simulink model "untitled2"  (R2018a)
settings: Solver=ode45  StartTime=0.0  StopTime=10  RelTol=1e-3
settings Model: Creator=HLY  LastModifiedBy=14223
settings CodeAppCC: StateflowObjectComments=on

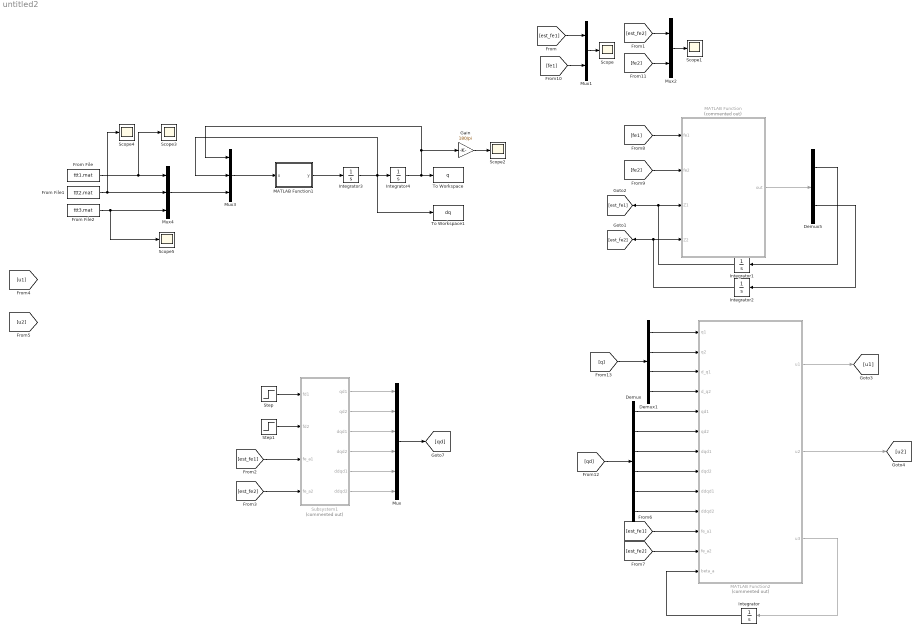
== system untitled2 ==
  Demux : Demux  Outputs=6
  Demux1 : Demux
  Demux5 : Demux  Outputs=[1;1]
  From File : FromFile  FileName=ttt1.mat  OutDataTypeStr=double
  From File1 : FromFile  FileName=ttt2.mat  OutDataTypeStr=double
  From File2 : FromFile  FileName=ttt3.mat  OutDataTypeStr=double
  Gain : Gain  Gain=180/pi
  Integrator : Integrator
  Integrator1 : Integrator
  Integrator2 : Integrator
  Integrator3 : Integrator  InitialCondition=[0 0 0]
  Integrator4 : Integrator  InitialCondition=[0 0 0]
  MATLAB Function : MATLAB Function  Commented=on  TreatAsAtomicUnit=on
  MATLAB Function1 : MATLAB Function  TreatAsAtomicUnit=on
  MATLAB Function2 : MATLAB Function  Commented=on  TreatAsAtomicUnit=on
  Mux : Mux  Inputs=6
  Mux1 : Mux  Inputs=2
  Mux2 : Mux  Inputs=2
  Mux3 : Mux  Inputs=3
  Mux4 : Mux  Inputs=3
  Scope{,1..5} (6 alike) : Scope
  Step : Step  After=10  SampleTime=0
  Step1 : Step  After=10  SampleTime=0
  Subsystem1 : Subsystem  Commented=on
  To Workspace : ToWorkspace  VariableName=q  SampleTime=-1
  To Workspace1 : ToWorkspace  VariableName=dq  SampleTime=-1
  wires:
  MATLAB Function/1(out) -> Demux5/1
  Demux5/1 -> Integrator1/1
  Demux5/2 -> Integrator2/1
  [est_fe1] -> Mux1/1
  [est_fe2] -> Mux2/1
  Mux1/1 -> Scope/1
  Mux2/1 -> Scope1/1
  MATLAB Function2/1(u1) -> [u1]
  MATLAB Function2/2(u2) -> [u2]
  Integrator/1 -> MATLAB Function2/13(beta_a)
  MATLAB Function2/3(u3) -> Integrator/1
  Integrator1/1 -> MATLAB Function/3(Z1), [est_fe1]
  Integrator2/1 -> MATLAB Function/4(Z2), [est_fe2]
  Step/1 -> Subsystem1/1(fd1)
  Step1/1 -> Subsystem1/2(fd2)
  [est_fe1] -> Subsystem1/3(fe_a1)
  [est_fe2] -> Subsystem1/4(fe_a2)
  [est_fe1] -> MATLAB Function2/11(fe_a1)
  [est_fe2] -> MATLAB Function2/12(fe_a2)
  [fe2] -> MATLAB Function/2(fe2)
  [fe1] -> MATLAB Function/1(fe1)
  [fe1] -> Mux1/2
  [fe2] -> Mux2/2
  Mux/1 -> [qd]
  Subsystem1/1(qd1) -> Mux/1
  Subsystem1/2(qd2) -> Mux/2
  Subsystem1/3(dqd1) -> Mux/3
  Subsystem1/4(dqd2) -> Mux/4
  Subsystem1/5(ddqd1) -> Mux/5
  Subsystem1/6(ddqd2) -> Mux/6
  Demux/1 -> MATLAB Function2/5(qd1)
  Demux/2 -> MATLAB Function2/6(qd2)
  Demux/3 -> MATLAB Function2/7(dqd1)
  Demux/4 -> MATLAB Function2/8(dqd2)
  Demux/5 -> MATLAB Function2/9(ddqd1)
  Demux/6 -> MATLAB Function2/10(ddqd2)
  [qd] -> Demux/1
  [q] -> Demux1/1
  Demux1/4 -> MATLAB Function2/4(d_q2)
  Demux1/1 -> MATLAB Function2/1(q1)
  Demux1/2 -> MATLAB Function2/2(q2)
  Demux1/3 -> MATLAB Function2/3(d_q1)
  Gain/1 -> Scope2/1
  From File1/1 -> Scope4/1, Mux4/2
  Mux3/1 -> MATLAB Function1/1(u)
  Mux4/1 -> Mux3/3
  From File2/1 -> Scope5/1, Mux4/3
  Integrator4/1 -> Gain/1, Mux3/1, To Workspace/1
  MATLAB Function1/1(y) -> Integrator3/1
  Integrator3/1 -> To Workspace1/1, Mux3/2, Integrator4/1
  From File/1 -> Scope3/1, Mux4/1

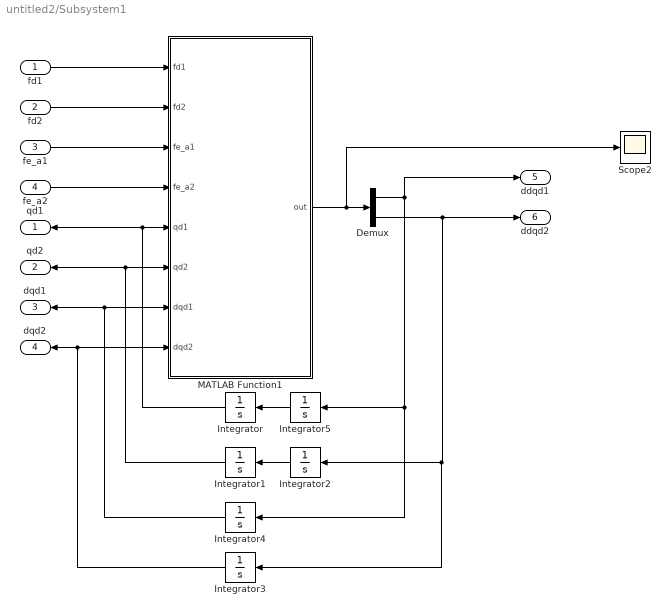
== system untitled2/Subsystem1 ==
  fd1 : Inport
  fd2 : Inport  Port=2
  fe_a1 : Inport  Port=3
  fe_a2 : Inport  Port=4
  Demux : Demux  Outputs=2
  Integrator : Integrator  InitialCondition=0.483
  Integrator1 : Integrator  InitialCondition=0.684
  Integrator{2..5} (4 alike) : Integrator
  MATLAB Function1 : MATLAB Function  TreatAsAtomicUnit=on
  Scope2 : Scope
  qd1 : Outport
  qd2 : Outport  Port=2
  dqd1 : Outport  Port=3
  dqd2 : Outport  Port=4
  ddqd1 : Outport  Port=5
  ddqd2 : Outport  Port=6
  wires:
  MATLAB Function1/1(out) -> Scope2/1, Demux/1
  fd1/1 -> MATLAB Function1/1(fd1)
  fd2/1 -> MATLAB Function1/2(fd2)
  fe_a1/1 -> MATLAB Function1/3(fe_a1)
  fe_a2/1 -> MATLAB Function1/4(fe_a2)
  Integrator/1 -> qd1/1, MATLAB Function1/5(qd1)
  Integrator5/1 -> Integrator/1
  Integrator2/1 -> Integrator1/1
  Integrator1/1 -> MATLAB Function1/6(qd2), qd2/1
  Integrator4/1 -> MATLAB Function1/7(dqd1), dqd1/1
  Integrator3/1 -> dqd2/1, MATLAB Function1/8(dqd2)
  Demux/1 -> Integrator5/1, Integrator4/1, ddqd1/1
  Demux/2 -> Integrator3/1, Integrator2/1, ddqd2/1

== matlab function untitled2/MATLAB Function1 ==
  data: u input; y output
function y = fcn(u)
a1=0.02;a2=0.475;a3=0.02;g=9.81;
q0=u(1);q1=u(2);q2=u(3);
dq0=u(4);dq1=u(5);dq2=u(6);
tol1=u(7);tol2=u(8);tol3=u(9);
I1xx=0;I1xy=0;I1xz=0;I1yyc=0;I1yz=0;I1zzc=0.5;
l1x=0.5*a1;l1y=0;l1z=0;
m1=12;
rlx=l1x/m1;
I1yy=m1*(rlx^2);%平行轴定理
I1zz=I1zzc+m1*(rlx^2);
I2xx=0;I2xy=0;I2xz=0;I2yyc=0;I2yz=0;I2zzc=0.2;
l2x=0.5*a2;l2y=0;l2z=0;
m2=8;
r2x=l2x/m2;
I2yy=m2*(r2x^2);
I2zz=I2zzc+m2*(r2x^2);
I3xx=0;I3xy=0;I3xz=0;I3yyc=0;I3yz=0;I3zzc=0.1;
l3x=0.5*a3;l3y=0;l3z=0;
m3=5;
r3x=l3x/m3;
I3yy=m3*(r3x^2);
I3zz=I3zzc+m3*(r3x^2);
F1s=97.26;F1v=96.14;F2s=1.03;F2v=65.03;F3s=33.43;F3v=19.3;
%F1s= 90;F1v=96.14;F2s=0;F2v=65.03;F3s=30;F3v=19.3;

 Xmin=[I1zz+I2yy+I3yy+m2*a1^2+m3*(a1^2+a2^2);I2xx-I2yy-m3*a2^2;I2xy;I2xz-a2*l3z;I2yz;I2zz+m3*a2^2;l2x+m3*a2;l2y;I3xx-I3yy;I3xy;I3xz;I3yz;I3zz;l3x;l3y;F1s;F1v;F2s;F2v;F3s;F3v];
 Xmin=[I1zz+I2yy+I3yy+m2*a1^2+m3*(a1^2+a2^2);I2xx-I2yy-m3*a2^2;I2xy;I2xz-a2*l3z;I2yz;I2zz+m3*a2^2;l2x+m3*a2;l2y;I3xx-I3yy;I3xy;I3xz;I3yz;I3zz;l3x;l3y;F1s;F1v;F2s;F2v;F3s;F3v];
 m11=Xmin(1)+(cos(q1)^2)*Xmin(2)-sin(2*q1)*Xmin(3)+2*a1*sin(q1)*Xmin(7)+2*a1*cos(q1)*Xmin(8)+(1/2+cos(2*q1+2*q2)/2)* Xmin(9)-sin(2*(q1+q2))*Xmin(10)+(a2.*cos(q2)+2*a1.*sin(q1+q2)-a2*cos(2*q1+q2))*Xmin(14)+(a2*sin(2*q1+q2)-a2*sin(q2)+2*a1*cos(q1+q2))*Xmin(15);
 m12=cos(q1)*Xmin(4)-sin(q1)*Xmin(5)+cos(q1+q2)*Xmin(11)-sin(q1+q2)*Xmin(12);
 m13=cos(q1+q2)*Xmin(11)-sin(q1+q2)*Xmin(12);
 m21=cos(q1)*Xmin(4)+cos(q1+q2)*Xmin(11)-sin(q1+q2)*Xmin(12);
 m22=Xmin(6)+Xmin(13)+2*a2.*cos(q2)*Xmin(14)- 2*a2*sin(q2)*Xmin(15);
 m23=Xmin(13)+a2*cos(q2)*Xmin(14)-2*a2*sin(q2)*Xmin(15);
 m31=cos(q1+q2)*Xmin(11)-sin(q1+q2)*Xmin(12);
 m32=Xmin(13)+a2*cos(q2)*Xmin(14)-a2*sin(q2)*Xmin(15);
 m33=Xmin(13);
 c1= -cos(q1).*2.*dq0.*dq1.*sin(q1)*Xmin(2)-2*dq0.*dq1.*cos(2*q1).*Xmin(3)-dq1.^2.*sin(q1)*Xmin(4)-(dq1.^2).*cos(q1)*Xmin(5)+2*a1*dq0.*dq1.*cos(q1)*Xmin(7)-2*a1*dq0.*dq1.*sin(q1)*Xmin(8)-(dq0.*dq1.*sin(2*q1+2*q2)+dq0.*dq2.*sin(2*q1+2*q2))*Xmin(9)-2*dq0.*(dq1+dq2).*cos(2*(q1+q2))*Xmin(10)-(sin(q1+q2).*dq1.^2+2*sin(q1+q2).*dq1.*dq2+sin(q1+q2).*dq2.^2)*Xmin(11)+...
    -((dq1+dq2).^2).*cos(q1+q2)*Xmin(12)+(2*a1*dq0.*dq1.*cos(q1+q2)+2*a1*dq0.*dq2.*cos(q1+q2)-a2*dq0.*dq2.*sin(q2)+2*a2*dq0.*dq1.*sin(2*q1+q2)+a2*dq0.*dq2.*sin(2*q1+q2))*Xmin(14)+(-2*a1*dq0.*dq1.*sin(q1+q2)-2*a1*dq0.*dq2.*sin(q1+q2)-a2*dq0.*dq2.*cos(q2)+2*a2*dq0.*dq1.*cos(2*q1+q2)+a2*dq0.*dq2.*cos(2*q1+q2))*Xmin(15);
 c2=(dq0.^2).*cos(q1).*sin(q1)*Xmin(2)+(dq0.^2).*cos(2*q1)*Xmin(3)-a1*(dq0.^2).*cos(q1)*Xmin(7)+a1*(dq0.^2).*sin(q1)*Xmin(8)+((dq0.^2).*sin(2*(q1+q2)))/2*Xmin(9)+(dq0.^2).*cos(2*(q1+q2))*Xmin(10)+(-a1*dq0.^2.*cos(q1+q2)-a2*dq2.^2.*sin(q2)-a2*dq0.^2.*sin(2*q1+q2)-2*a2*dq1.*dq2.*sin(q2))*Xmin(14)+(a1*dq0.^2.*sin(q1+q2)-a2*dq2.^2.*cos(q2)-a2*dq0.^2.*cos(2*q1+q2)-2*a2*dq1.*dq2.*cos(q2))*Xmin(15);
 c3=0.5*dq0.^2.*sin(2*(q1+q2))*Xmin(9)+dq0.^2.*cos(2*(q1+q2))*Xmin(10)+(cos(q2).*(a2*(-cos(q1)).*sin(q1).*dq0.^2-a1*dq0.^2.*cos(q1))-sin(q2).*(-a2.*(dq0.^2.*sin(q1).^2+dq1.^2)-a1*dq0.^2.*sin(q1)))*Xmin(14)+...
    +(-sin(q2).*(a2*(-cos(q1).*sin(q1).*dq0.^2)-a1*dq0.^2.*cos(q1))-cos(q2).*(-a2.*(dq0.^2.*sin(q1).^2+dq1.^2)-a1*dq0.^2.*sin(q1)))*Xmin(15);
 g1=0;
 g2=(-g*sin(q1)*Xmin(7)-g*cos(q1)*Xmin(8)-g*sin(q1+q2)*Xmin(14)-g*cos(q1+q2)*Xmin(15));
 g3=(-g*(sin(q1)*cos(q2)+sin(q2)*cos(q1))*Xmin(14)- g*(-sin(q1)*sin(q2)+cos(q1)*cos(q1))*Xmin(15));
 f1=sign(dq0)*Xmin(16)+dq0*Xmin(17);
 f2=sign(dq1)*Xmin(18)+dq1*Xmin(19);
 f3=sign(dq2)*Xmin(20)+dq2*Xmin(21);
 M=[m11,m12,m13;m21,m22,m23;m31,m32,m33];C=[c1;c2;c3];G=[g1;g2;g3];f=[f1;f2;f3];tol=[tol1;tol2;tol3];
 ddq=inv(M)*(tol-C-G-f);
 y=ddq;
end

== matlab function untitled2/MATLAB Function ==
  data: out output; fe1 input; fe2 input; Z1 input; Z2 input
function out=Est_contactforce(fe1,fe2,Z1,Z2)
L=[50 0;0 50];
Fe=[fe1;fe2];
%Fe=Ke*(X-Xe);
Z=[Z1;Z2];
dEst_Fe=L*(Fe-Z);
out=dEst_Fe;

== matlab function untitled2/MATLAB Function2 ==
  data: q1 input; q2 input; d_q1 input; d_q2 input; qd1 input; u1 output; qd2 input; dqd1 input; dqd2 input; ddqd1 input; ddqd2 input; fe_a1 input; u2 output; fe_a2 input; beta_a input; u3 output
function [u1,u2,u3] = fcn(q1,q2,d_q1,d_q2,qd1,qd2,dqd1,dqd2,ddqd1,ddqd2,fe_a1,fe_a2,beta_a)
l1=1;l2=0.8;j1=5;j2=5;m1=0.5;m2=1.5;
a11=(m1+m2)*l1^2+m2*l2^2+2*m2*l1*l2*cos(q2)+j1;
a12=m2*l2^2+m2*l1*l2*cos(q2);
a22=m2*l2^2+j2;
M=[a11,a12;a12,a22];
beta12=m2*l1*l2*sin(q2);
c1=-beta12*d_q1^2-2*beta12*d_q1*d_q2;
c2=beta12*d_q2^2;
C=[c1;c2];
gama1=(m1+m2)*l2*cos(q2)+m2*l2*cos(q1+q2);
gama2=m2*l2*cos(q1+q2);
g=[gama1;gama2];
p1=l1*cos(q1)+l2*cos(q1+q2);
p2=l1*sin(q1)+l2*sin(q1+q2);
J=[-p2,-l2*sin(q1+q2);p1,l2*cos(q1+q2)];
q=[q1;q2];dq=[d_q1;d_q2];
qd=[qd1;qd2];dqd=[dqd1;dqd2];
ddqd=[ddqd1;ddqd2];
fe_a=[fe_a1;fe_a2];
e=qd-q;de=dqd-dq;
c=[20,0;0,20];k=[100,0;0,100];
s=c*e+de;
gama=[0.05,0;0,0.05];
%beta_a=norm(J*s,2)*gama;
tol=J'*fe_a+C+g+M*(c*de+ddqd+k*s)+J*beta_a*[sign(s(1));sign(s(2))];
%out=tol;
u1=tol(1);u2=tol(2);u3=norm(J*s,2)*gama;

== matlab function untitled2/Subsystem1/MATLAB Function1 ==
  data: fd1 input; fd2 input; fe_a1 input; out output; fe_a2 input; qd1 input; qd2 input; dqd1 input; dqd2 input
function out = fcn(fd1,fd2,fe_a1,fe_a2,qd1,qd2,dqd1,dqd2)
l1=1;l2=0.8;
pd1=l1*cos(qd1)+l2*cos(qd1+qd2);
pd2=l1*sin(qd1)+l2*sin(qd1+qd2);
dpd1=-l1*sin(qd1)*dqd1-l2*sin(qd1+qd2)*(dqd1+dqd2);
dpd2=l1*cos(qd1)*dqd1+l2*cos(qd1+qd2)*(dqd1+dqd2);
J=[-pd2,-l2*sin(qd1+qd2);pd1,l2*cos(qd1+qd2)];
dJ=[-dpd2,-l2*cos(qd1+qd2)*(dqd1+dqd2);dpd1,-12*sin(qd1+qd2)*(dqd1+dqd2)];
fd=[fd1;fd2];fe_a=[fe_a1;fe_a2];
M1=[20,0;0,20];B1=[1000,0;0,1000];
dqd=[dqd1;dqd2];
ddqd=inv(J)*inv(M1)*(fd-fe_a-(M1*dJ+B1*J)*dqd);
%dqd1=dqd(1);dqd2=dqd(2);
out=ddqd;
